simulink model "ex_han"  (Simulink 8.9)
settings: Solver=FixedStepAuto  StartTime=0.0  StopTime=15.0  FixedStep=0.0001  RelTol=1e-3
settings Model: SuppressorTable=22 serialization::archive 11 0 6 0 0 0 11 0  Creator=rastronaut  LastModifiedBy=rastronaut
settings DataIOCC: LimitDataPoints=off  SaveFormat=Dataset  SignalLoggingSaveFormat=Dataset
settings OptimizationCC: LifeSpan=auto
settings DebuggingCC: UnderspecifiedInitializationDetection=Simplified  MergeDetectMultiDrivingBlocksExec=error  FcnCallInpInsideContextMsg=error  StateNameClashWarn=none  SFUnexpectedBacktrackingDiag=error  SFNoUnconditionalDefaultTransitionDiag=error  SFExecutionAtInitializationDiag=warning
settings HardwareCC: ProdBitPerPointer=64  ProdBitPerSizeT=64  ProdBitPerPtrDiffT=64  ProdLargestAtomicFloat=Float  ProdIntDivRoundTo=Zero  ProdEndianess=LittleEndian  ProdWordSize=64  ProdHWDeviceType=Intel->x86-64 (Windows64)
settings ModelReferenceCC: PropagateSignalLabelsOutOfModel=on
settings GRTTargetCC: TargetLangStandard=C99 (ISO)  GeneratePreprocessorConditionals=Use local settings  CombineOutputUpdateFcns=on  GRTInterface=off
settings ConfigComp: CovMetricSettings=dwe  CovHtmlReporting=off  CovSaveCumulativeToWorkspaceVar=off  CovSaveSingleToWorkspaceVar=off  CovExternalEMLEnable=on

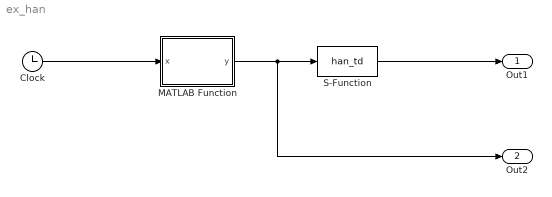
== system ex_han ==
  Clock : Clock
  MATLAB Function : MATLAB Function  TreatAsAtomicUnit=on
  S-Function : S-Function  FunctionName=han_td  Parameters=r, h, T  SFunctionDeploymentMode=off  EnableBusSupport=off
  Out1 : Outport
  Out2 : Outport  Port=2
  wires:
  MATLAB Function/1(y) -> Out2/1, S-Function/1
  S-Function/1 -> Out1/1
  Clock/1 -> MATLAB Function/1(x)

== matlab function MATLAB Function ==
  data: x input double; y output double
function y=han_fun(x)
if x<=2*pi, y=sin(x);                   % sinusoidal wave in the first period
elseif x<=2.5*pi, y=2*(x-2*pi)/pi;      % followed by triangular waves
elseif x<=3.5*pi, y=1-2*(x-2.5*pi)/pi;
elseif x<=4*pi, y=-2+2*(x-3*pi)/pi;
else y = 0; end
